simulink subsystem "controller"  (R2021a)
settings: Solver=VariableStepAuto  StartTime=0.0  StopTime=10.0  RelTol=1e-3
settings Model: Creator=Sirius  LastModifiedBy=Sirius

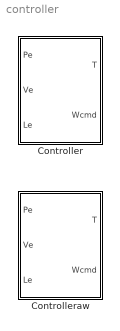
== system controller ==
  Controller : Subsystem
  Controlleraw : Subsystem

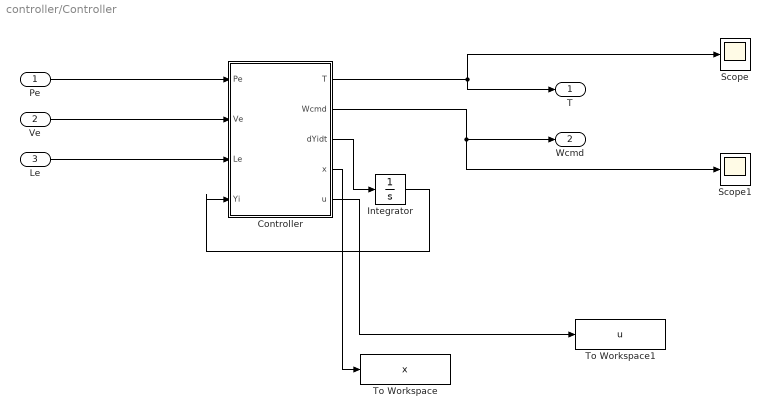
== system controller/Controller ==
  Pe : Inport
  Ve : Inport  Port=2
  Le : Inport  Port=3
  Controller : MATLAB Function  TreatAsAtomicUnit=on
  Integrator : Integrator  InitialCondition=[0;0;0;0]
  Scope : Scope
  Scope1 : Scope
  To Workspace : ToWorkspace  VariableName=x  SaveFormat=Timeseries  SampleTime=-1
  To Workspace1 : ToWorkspace  VariableName=u  SaveFormat=Timeseries  SampleTime=-1
  T : Outport  VectorParamsAs1DForOutWhenUnconnected=off
  Wcmd : Outport  Port=2  VectorParamsAs1DForOutWhenUnconnected=off
  wires:
  Controller/1(T) -> T/1, Scope/1
  Controller/2(Wcmd) -> Wcmd/1, Scope1/1
  Controller/3(dYidt) -> Integrator/1
  Integrator/1 -> Controller/4(Yi)
  Pe/1 -> Controller/1(Pe)
  Ve/1 -> Controller/2(Ve)
  Le/1 -> Controller/3(Le)
  Controller/4(x) -> To Workspace/1
  Controller/5(u) -> To Workspace1/1

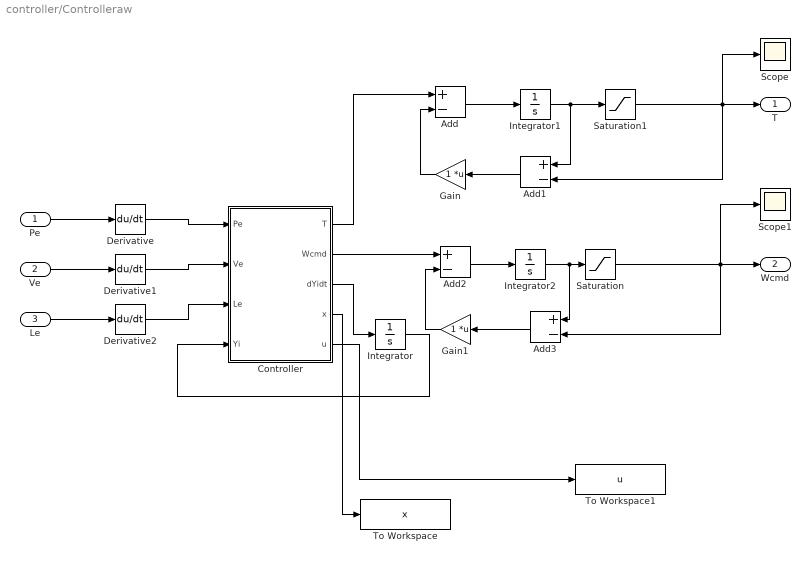
== system controller/Controlleraw ==
  Pe : Inport
  Ve : Inport  Port=2
  Le : Inport  Port=3
  Add{,1..3} (4 alike) : Sum  Inputs=+-
  Controller : MATLAB Function  TreatAsAtomicUnit=on
  Derivative : Derivative
  Derivative1 : Derivative
  Derivative2 : Derivative
  Gain : Gain  Multiplication=Matrix(K*u)
  Gain1 : Gain  Multiplication=Matrix(K*u)
  Integrator : Integrator  InitialCondition=[0;0;0;0]
  Integrator1 : Integrator
  Integrator2 : Integrator
  Saturation : Saturate  UpperLimit=[5;5;5]  LowerLimit=-[5;5;5]
  Saturation1 : Saturate  UpperLimit=20  LowerLimit=-20
  Scope : Scope
  Scope1 : Scope
  To Workspace : ToWorkspace  VariableName=x  SaveFormat=Timeseries  SampleTime=-1
  To Workspace1 : ToWorkspace  VariableName=u  SaveFormat=Timeseries  SampleTime=-1
  T : Outport  VectorParamsAs1DForOutWhenUnconnected=off
  Wcmd : Outport  Port=2  VectorParamsAs1DForOutWhenUnconnected=off
  wires:
  Controller/3(dYidt) -> Integrator/1
  Integrator/1 -> Controller/4(Yi)
  Controller/4(x) -> To Workspace/1
  Controller/5(u) -> To Workspace1/1
  Pe/1 -> Derivative/1
  Derivative/1 -> Controller/1(Pe)
  Ve/1 -> Derivative1/1
  Derivative1/1 -> Controller/2(Ve)
  Le/1 -> Derivative2/1
  Derivative2/1 -> Controller/3(Le)
  Controller/1(T) -> Add/1
  Integrator1/1 -> Add1/1, Saturation1/1
  Add/1 -> Integrator1/1
  Gain/1 -> Add/2
  Saturation1/1 -> Add1/2, Scope/1, T/1
  Add2/1 -> Integrator2/1
  Integrator2/1 -> Add3/1, Saturation/1
  Add1/1 -> Gain/1
  Controller/2(Wcmd) -> Add2/1
  Saturation/1 -> Add3/2, Scope1/1, Wcmd/1
  Add3/1 -> Gain1/1
  Gain1/1 -> Add2/2

== matlab function controller/Controlleraw/Controller ==
  data: Pe input; T output; Ve input; Le input; Wcmd output; Ki parameter; Yi input; dYidt output; x output; u output
function [T,Wcmd,dYidt,x,u]=Controller(Pe,Ve,Le,Ki,Yi)
x=[Pe;Ve;Le;Yi];
u=-Ki*x;
T=u(1);
Wcmd=u(2:4);
dYidt=[Pe;Le(3)];
end

== matlab function controller/Controller/Controller ==
  data: Pe input; T output; Ve input; Le input; Wcmd output; Ki parameter; Yi input; dYidt output; x output; u output
function [T,Wcmd,dYidt,x,u]=Controller(Pe,Ve,Le,Ki,Yi)
x=[Pe;Ve;Le;Yi];
u=-Ki*x;
T=u(1);
Wcmd=u(2:4);
dYidt=[Pe;Le(3)];
end
